simulink model "VehicleThermalSystemSizing"  (R2023b)
settings: Solver=daessc  StartTime=0  StopTime=600  FixedStep=0.2  MaxStep=1  RelTol=1e-3  AbsTol=1e-3
undefined symbols (not defined in the file): air_density, bulb, cabin_H, cabin_L, cabin_W, coolant_pipe_D, coolant_T_init, coolant_tank_volume, CoolingPower_kW, door_or_window_area, duct_W, evap_superheat_temp, inlet, pump_speed_max, refrigerant_massflowrate, RPM_Compressor_nominal, RPM_CondFan, RPM_EvapFan, T_cabin_init, T_set, tube_D, VolFlowrate_CondenserFan, VolFlowRate_CoolantRadiatorFan, VolFlowRate_EvapFan
libraries: fl_lib x128, nesl_utility x45, SimscapeFluids_lib x16, simulink_extras x9
(part 1 of 4)
Description:
  | Refrigeration Cycle (Air Conditioning)
settings Model: Creator=The MathWorks, Inc.  LastModifiedBy=fnae
settings SolverCC: AutoScaleAbsTol=off  AlgebraicLoopSolver=TrustRegion  MaxZcPerStep=1
settings DataIOCC: SaveFormat=StructureWithTime  ReturnWorkspaceOutputs=off
settings OptimizationCC: BlockReduction=off  BufferReuse=off  ReuseModelBlockBuffer=off
settings DebuggingCC: AlgebraicLoopMsg=none  SymbolicDimsDataTypeCodeGenerationDiagnostic=none
settings ModelReferenceCC: EnableRefExpFcnMdlSchedulingChecks=on
settings SFSimCC: CustomCodeUndefinedFunction=UseInterfaceOnly
settings RTWCC: DLArmComputeVersion=19.05
settings SimscapeCC: SimscapeLogType=all  SimscapeLogSimulationStatistics=on  SimscapeLogName=simlog_refrigeration  SimscapeLogLimitData=off  SimscapeLogDataHistory=10000  SimscapeOperatingPoint=operPoint
settings ExplorerConfigSet: SimMechanicsOpenEditorOnUpdate=off

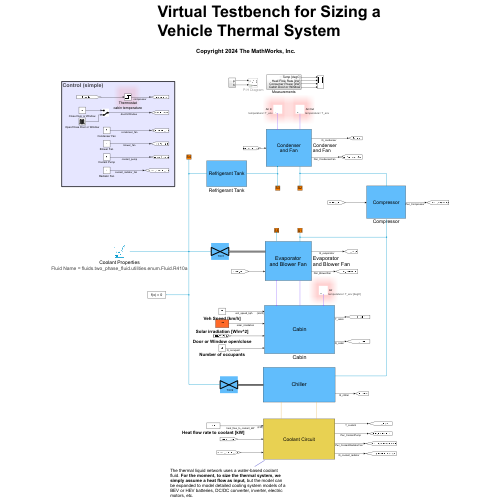
[thumbnail: Simulink's stored preview of the top-level diagram]
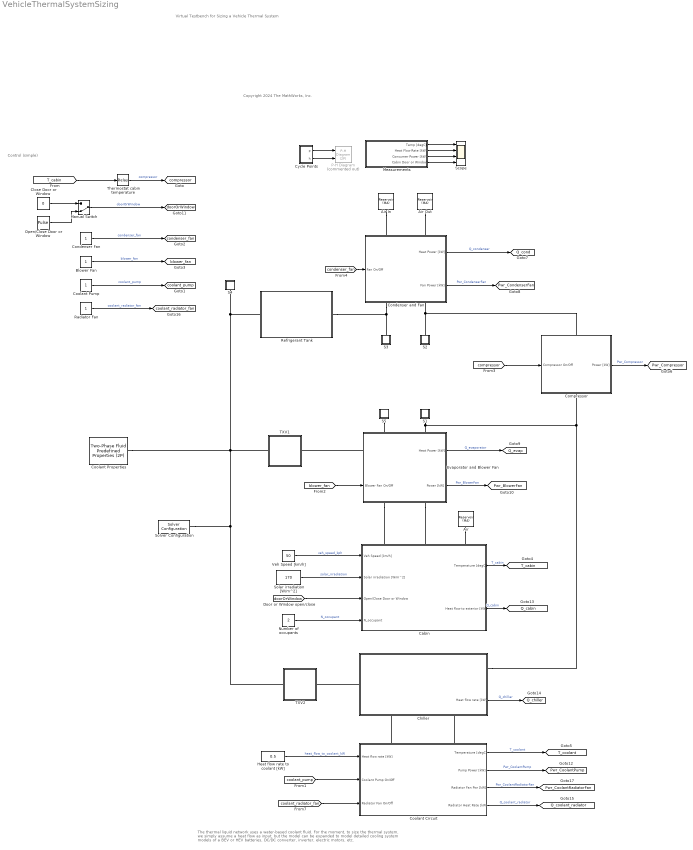
== system VehicleThermalSystemSizing ==
  note: The thermal liquid network uses a water-based coolant fluid. For the moment, to size the thermal system, we simply assume a heat flow as input, but the model can be expanded to model detailed cooling system models of a BEV or HEV batteries, DC/DC converter, inverter, electric motors, etc.
  note: Control (simple)
  note: Virtual Testbench for Sizing a Vehicle Thermal System
  note: Copyright 2024 The MathWorks, Inc.
  Air : fl_lib/Moist Air/Elements/Reservoir (MA)  pressure_spec=foundation.enum.pressure_spec.specified  reservoir_pressure=0.101325 MPa  temperature_spec=foundation.enum.temperature_spec.specified  reservoir_temperature=T_env degC  moisture_spec=foundation.enum.moisture_spec.relative_humidity  reservoir_RH=0.5  reservoir_x_w=0.01  reservoir_y_w=0.01  reservoir_HR=0.01  reservoir_Tw=287 K  trace_gas_spec=foundation.enum.trace_gas_spec.mole_fraction  reservoir_x_g=0.001  reservoir_y_g=0  RH_ws=1  area_A=duct_W^2 m^2
      settings: AttributesFormatString=temperature= %<reservoir_temperature> [%<reservoir_temperature_unit>]
  Air In : fl_lib/Moist Air/Elements/Reservoir (MA)  pressure_spec=foundation.enum.pressure_spec.specified  reservoir_pressure=0.101325 MPa  temperature_spec=foundation.enum.temperature_spec.specified  reservoir_temperature=T_env degC  moisture_spec=foundation.enum.moisture_spec.relative_humidity  reservoir_RH=0.5  reservoir_x_w=0.01  reservoir_y_w=0.01  reservoir_HR=0.01  reservoir_Tw=287 K  trace_gas_spec=foundation.enum.trace_gas_spec.mole_fraction  reservoir_x_g=0.001  reservoir_y_g=0  RH_ws=1  area_A=duct_W^2 m^2
      settings: AttributesFormatString=temperature= %<reservoir_temperature>
  Air Out : fl_lib/Moist Air/Elements/Reservoir (MA)  pressure_spec=foundation.enum.pressure_spec.specified  reservoir_pressure=0.101325 MPa  temperature_spec=foundation.enum.temperature_spec.specified  reservoir_temperature=T_env degC  moisture_spec=foundation.enum.moisture_spec.relative_humidity  reservoir_RH=0.5  reservoir_x_w=0.01  reservoir_y_w=0.01  reservoir_HR=0.01  reservoir_Tw=287 K  trace_gas_spec=foundation.enum.trace_gas_spec.mole_fraction  reservoir_x_g=0.001  reservoir_y_g=0  RH_ws=1  area_A=duct_W^2 m^2
      settings: AttributesFormatString=temperature= %<reservoir_temperature>
  Blower Fan : Constant  SampleTime=1
  Cabin : Subsystem
      settings: PortSchema="{\"entries\":[{\"content\":{\"sides\":[{\"content\":{\"connectorIds\":[\"In1\",\"In2\",\"In3\",\"In4\"]},\"type\":\"ConnectorPlacement.EquallySpacedRectSide\",\"uuid\":\"5cf57e4f-975f-4b0b-a8e8-bf86758a11fa\"},{\"content\":{\"connectorIds\":[\"Out1\",\"Out2\"],\"side\":\"RIGHT\"},\"type\":\"ConnectorPlacement.EquallySpacedRectSide\",\"uuid\":\"7f477a27-3a34-4ed6-85c3-331630c97133\"},{\"content\":{\"connectorIds\":[\"LConn1\",\"LConn2\",\"LConn3\"],\"side\":\"TOP\"},\"type\":\"ConnectorPlacement.EquallySpacedRectSide\",\"uuid\":\"743b5c17-84cf-4a2e-818e-c1a69eb195e5\"}]},\"type\":\"ConnectorPlacement.EquallySpacedConnector\",\"uuid\":\"4a6d6dd0-79df-4460-8879-70a258476fa5\"}],\"packageUris\":[\"http://schema.mathworks.com/mf0/Connector/R2020b\"],\"version\":\"1.0\"}"
      mask Display: disp(get_param(gcb, 'Name'));
  Chiller : Subsystem  Tag=PublishSubsystem
      settings: PortSchema="{\"entries\":[{\"content\":{\"sides\":[{\"content\":{\"connectorIds\":[\"Out1\",\"LConn1\"]},\"type\":\"ConnectorPlacement.EquallySpacedRectSide\",\"uuid\":\"684495fe-43ac-42d2-91f9-c1083f68d635\"},{\"content\":{\"connectorIds\":[\"RConn1\"],\"side\":\"RIGHT\"},\"type\":\"ConnectorPlacement.EquallySpacedRectSide\",\"uuid\":\"acb3d27a-41e1-4bfe-a4d6-36d5666e4ba3\"},{\"content\":{\"connectorIds\":[\"LConn2\",\"LConn3\"],\"side\":\"TOP\"},\"type\":\"ConnectorPlacement.EquallySpacedRectSide\",\"uuid\":\"cdadeb40-472c-4edb-91b8-a2216ea85c99\"},{\"content\":{\"side\":\"BOTTOM\"},\"type\":\"ConnectorPlacement.EquallySpacedRectSide\",\"uuid\":\"46a4312c-e637-44ea-bfb3-e887da9d9904\"}]},\"type\":\"ConnectorPlacement.EquallySpacedConnector\",\"uuid\":\"20e25167-e167-414a-8c66-12b35ae5ef5e\"}],\"packageUris\":[\"http://schema.mathworks.com/mf0/Connector/R2020b\"],\"version\":\"1.0\"}"
      mask Display: disp(get_param(gcb, 'Name'));
  Close Door or Window : Constant  Value=0  SampleTime=1
  Compressor : Subsystem
      settings: PortSchema="{\"entries\":[{\"content\":{\"sides\":[{\"content\":{\"connectorIds\":[\"LConn1\"]},\"type\":\"ConnectorPlacement.EquallySpacedRectSide\",\"uuid\":\"87497da4-7fcd-4c39-9d14-dd80365934db\"},{\"content\":{\"connectorIds\":[\"RConn1\"],\"side\":\"RIGHT\"},\"type\":\"ConnectorPlacement.EquallySpacedRectSide\",\"uuid\":\"c29b3d2b-7130-4a2f-8dcb-58b301edb84d\"},{\"content\":{\"connectorIds\":[\"In1\"],\"side\":\"TOP\"},\"type\":\"ConnectorPlacement.EquallySpacedRectSide\",\"uuid\":\"6b0e1579-3829-4056-a1f0-26424a36bca1\"},{\"content\":{\"connectorIds\":[\"Out1\"],\"side\":\"BOTTOM\"},\"type\":\"ConnectorPlacement.EquallySpacedRectSide\",\"uuid\":\"6b49380d-e724-4e3a-86e0-6bc21724e354\"}]},\"type\":\"ConnectorPlacement.EquallySpacedConnector\",\"uuid\":\"16d6c8a7-8265-44ec-91d1-631bbb83e0af\"}],\"packageUris\":[\"http://schema.mathworks.com/mf0/Connector/R2020b\"],\"version\":\"1.0\"}"
      mask Display: disp(get_param(gcb, 'Name'));
  Condenser and Fan : Subsystem
      settings: PortSchema="{\"entries\":[{\"content\":{\"sides\":[{\"content\":{\"connectorIds\":[\"LConn1\",\"LConn2\"]},\"type\":\"ConnectorPlacement.EquallySpacedRectSide\",\"uuid\":\"94f743b0-016e-4f6c-ba37-cd5c9e5decb1\"},{\"content\":{\"connectorIds\":[\"RConn1\",\"RConn2\"],\"side\":\"RIGHT\"},\"type\":\"ConnectorPlacement.EquallySpacedRectSide\",\"uuid\":\"4e78d493-e8a5-489f-9c9b-6c9134237572\"},{\"content\":{\"connectorIds\":[\"In1\"],\"side\":\"TOP\"},\"type\":\"ConnectorPlacement.EquallySpacedRectSide\",\"uuid\":\"0b95dc75-9fe3-4b9e-8dc0-c99924a5b683\"},{\"content\":{\"connectorIds\":[\"Out1\",\"Out2\"],\"side\":\"BOTTOM\"},\"type\":\"ConnectorPlacement.EquallySpacedRectSide\",\"uuid\":\"eea3e702-1cf4-4504-9501-89c4531d7134\"}]},\"type\":\"ConnectorPlacement.EquallySpacedConnector\",\"uuid\":\"0b0f7158-6d74-402a-9204-25c9a3fd4099\"}],\"packageUris\":[\"http://schema.mathworks.com/mf0/Connector/R2020b\"],\"version\":\"1.0\"}"
      mask Display: disp(get_param(gcb, 'Name'));
  Condenser Fan : Constant  SampleTime=1
  Coolant Circuit : Subsystem
      settings: PortSchema="{\"entries\":[{\"content\":{\"sides\":[{\"content\":{\"connectorIds\":[\"In1\",\"In2\",\"In3\"]},\"type\":\"ConnectorPlacement.EquallySpacedRectSide\",\"uuid\":\"61b3bd2b-efba-48b8-bc1e-7d5fd1f93ea8\"},{\"content\":{\"connectorIds\":[\"Out1\",\"Out2\",\"Out3\",\"Out4\"],\"side\":\"RIGHT\"},\"type\":\"ConnectorPlacement.EquallySpacedRectSide\",\"uuid\":\"116770ca-4665-4fbe-8ef7-14ad65bf6363\"},{\"content\":{\"connectorIds\":[\"LConn1\",\"LConn2\"],\"side\":\"TOP\"},\"type\":\"ConnectorPlacement.EquallySpacedRectSide\",\"uuid\":\"8588f2a2-4124-40f5-9c68-b1b3344e047c\"}]},\"type\":\"ConnectorPlacement.EquallySpacedConnector\",\"uuid\":\"af351b75-e118-4ad1-8604-555a25a7fec0\"}],\"packageUris\":[\"http://schema.mathworks.com/mf0/Connector/R2020b\"],\"version\":\"1.0\"}"
      mask Display: disp(get_param(gcb, 'Name'));
  Coolant Properties : SimscapeFluids_lib/Two-Phase Fluid/Utilities/Two-Phase Fluid Predefined Properties (2P)  fluid=fluids.two_phase_fluid.utilities.enum.Fluid.R410a  p_atm=0.101325 MPa  properties_range_check=simscape.enum.assert.action.error  q_rev=0.01 Pa
      settings: AttributesFormatString=Fluid Name = %<fluid>
  Coolant Pump : Constant  SampleTime=1
  Cycle Points : Subsystem
  Evaporator and Blower Fan : Subsystem
      settings: PortSchema="{\"entries\":[{\"content\":{\"sides\":[{\"content\":{\"connectorIds\":[\"LConn1\",\"LConn2\"]},\"type\":\"ConnectorPlacement.EquallySpacedRectSide\",\"uuid\":\"94f743b0-016e-4f6c-ba37-cd5c9e5decb1\"},{\"content\":{\"connectorIds\":[\"RConn1\",\"RConn2\"],\"side\":\"RIGHT\"},\"type\":\"ConnectorPlacement.EquallySpacedRectSide\",\"uuid\":\"4e78d493-e8a5-489f-9c9b-6c9134237572\"},{\"content\":{\"connectorIds\":[\"LConn3\",\"In1\"],\"side\":\"TOP\"},\"type\":\"ConnectorPlacement.EquallySpacedRectSide\",\"uuid\":\"0b95dc75-9fe3-4b9e-8dc0-c99924a5b683\"},{\"content\":{\"connectorIds\":[\"Out1\",\"Out2\"],\"side\":\"BOTTOM\"},\"type\":\"ConnectorPlacement.EquallySpacedRectSide\",\"uuid\":\"3125a7ac-4364-4843-9f9a-28cc842c280f\"}]},\"type\":\"ConnectorPlacement.EquallySpacedConnector\",\"uuid\":\"0b0f7158-6d74-402a-9204-25c9a3fd4099\"}],\"packageUris\":[\"http://schema.mathworks.com/mf0/Connector/R2020b\"],\"version\":\"1.0\"}"
      mask Display: disp(get_param(gcb, 'Name'));
  Heat flow rate to coolant [kW] : Constant  Value=0.5  SampleTime=1
  Manual Switch : ManualSwitch  CurrentSetting=0
  Measurements : Subsystem
  Number of occupants : Constant  Value=2  SampleTime=1
  Open/Close Door or Window : DiscretePulseGenerator  PulseType=Time based  Period=300  PulseWidth=5
  P-H Diagram : SimscapeFluids_lib/Two-Phase Fluid/Utilities/P-H Diagram (2P)  Commented=on
  Radiator Fan : Constant  SampleTime=1
  Refrigerant Tank : Subsystem
      mask Display: disp(get_param(gcb, 'Name'));
  S1 : Subsystem
      mask Display: disp(get_param(gcb, 'Name'))
  S2 : Subsystem
      mask Display: disp(get_param(gcb, 'Name'))
  S3 : Subsystem
      settings: PortSchema="{\"entries\":[{\"content\":{\"sides\":[{\"content\":{\"connectorIds\":[]},\"type\":\"ConnectorPlacement.EquallySpacedRectSide\",\"uuid\":\"16f002de-4636-401c-8be6-20698decbc91\"},{\"content\":{\"connectorIds\":[],\"side\":\"RIGHT\"},\"type\":\"ConnectorPlacement.EquallySpacedRectSide\",\"uuid\":\"76477188-11a3-4efa-a92e-0d269d480ac3\"},{\"content\":{\"connectorIds\":[],\"side\":\"TOP\"},\"type\":\"ConnectorPlacement.EquallySpacedRectSide\",\"uuid\":\"05fe64e4-9858-4712-a671-6ec27cab8615\"},{\"content\":{\"connectorIds\":[\"RConn1\"],\"side\":\"BOTTOM\"},\"type\":\"ConnectorPlacement.EquallySpacedRectSide\",\"uuid\":\"ddad7bbe-c900-450c-9863-e8fdc2274286\"}]},\"type\":\"ConnectorPlacement.EquallySpacedConnector\",\"uuid\":\"12bdef6d-66b8-4c10-9167-065994fcb3b8\"}],\"packageUris\":[\"http://schema.mathworks.com/mf0/Connector/R2020b\"],\"version\":\"1.0\"}"
      mask Display: disp(get_param(gcb, 'Name'))
  S4 : Subsystem
      mask Display: disp(get_param(gcb, 'Name'))
  S5 : Subsystem
      mask Display: disp(get_param(gcb, 'Name'))
  Scope : Scope  NumInputPorts=4
  Solar irradiation [W/m^2] : Constant  Value=170
  Solver Configuration : nesl_utility/Solver Configuration  PhysicalDomain=network_engine_domain  SubClassName=solver  LeftPortType=input  RightPortType=generic  Tones=[]  Harmonics=[]  SimulateNoise=off  Profile=off  UseLocalSampling=off  EnableSwitchedLinearOptims=on  FrequencyDomain=off  UseCCode=off  RelTol=0.001  AbsTol=0.001  MinStep=1e-09  ToWorkspace=off  RevertToSquareIcSolve=off  NumHomotopyIterations=100  PhasorMode=off  PhasorModeNumHarmonics=1  ConsistencySolver=NEWTON_XTOL_AFTER_FTOL  IndexReductionMethod=DerivativeReplacement  DoDC=off  ResidualTolerance=1e-6  ConsistencyTolSource=GLOBAL  ConsistencyAbsTol=0.001  ConsistencyRelTol=0.001  ConsistencyTolFactor=0.001  UseLocalSolver=off  LocalSolverChoice=NE_BACKWARD_EULER_ADVANCER  ResolveIndetEquations=on  FunctionEvalNumThread=1  LocalSolverSampleTime=0.01  DoFixedCost=off  MaxNonlinIter=100  MaxModeIter=10  ComputeImpulses=off  ImpulseIterations=2  LinearAlgebra=auto  LinearAlgebraNumThread=0  EquationFormulation=NE_TIME_EF  DelaysMemoryBudget=1024  AutomaticFiltering=on  FilteringTimeConstant=0.001  PartitionStorageMethod=AS_NEEDED  PartitionMemoryBudget=1024  PartitionMethod=ROBUST  MultibodyUseLocalSolver=off  MultibodyLocalSolverChoice=ODE1  MultibodyLocalSolverSampleTime=0.001
  TXV1 : Subsystem  Tag=PublishSubsystem
      mask Display:
      | color('white')
      | plot(100, 100)
      | plot(-100, -100)
      | color('black')
      | 
      | plot([0 -100 -100 0], [0 50 -50 0])
      | plot([0 100 100 0], [0 50 -50 0])
      | 
      | text(-50,60,get_param(gcb, 'Name'))
  TXV2 : Subsystem  Tag=PublishSubsystem
      mask Display:
      | color('white')
      | plot(100, 100)
      | plot(-100, -100)
      | color('black')
      | 
      | plot([0 -100 -100 0], [0 50 -50 0])
      | plot([0 100 100 0], [0 50 -50 0])
      | 
      | text(-50,60,get_param(gcb, 'Name'))
  Thermostat cabin temperature : Relay  OnSwitchValue=T_set + 1  OffSwitchValue=T_set  ZeroCross=off
  Veh Speed [km/h] : Constant  Value=50  SampleTime=1
  tag scope: Pwr_BlowerFan=global, Pwr_Compressor=global, Pwr_CondenserFan=global, Pwr_CoolantPump=global, Pwr_CoolantRadiatorFan=global, Q_cabin=global, Q_chiller=global, Q_cond=global, Q_coolant_radiator=global, Q_evap=global, T_cabin=global, T_coolant=global, blower_fan=global, compressor=global, condenser_fan=global, coolant_pump=global, coolant_radiator_fan=global, doorOrWindow=global
  wires:
  Cycle Points/1(p) -> P-H Diagram/1
  Cycle Points/2(h) -> P-H Diagram/2
  Measurements/1(Temp [degC]) -> Scope/1
  Measurements/2(Heat Flow Rate [kW]) -> Scope/2
  Measurements/3(Consumer Power [kW]) -> Scope/3
  Measurements/4(Cabin Door or Window) -> Scope/4
  [T_cabin] -> Thermostat cabin temperature/1
  [condenser_fan] -> Condenser and Fan/1(Fan On/Off)
  Condenser Fan/1 -> [condenser_fan]  "condenser_fan"
  [compressor] -> Compressor/1(Compressor On/Off)
  Blower Fan/1 -> [blower_fan]  "blower_fan"
  [blower_fan] -> Evaporator and Blower Fan/1(Blower Fan On/Off)
  Veh Speed [km/h]/1 -> Cabin/1(Veh Speed [km/h])  "veh_speed_kph"
  Solar irradiation [W/m^2]/1 -> Cabin/2(Solar irradiation [W/m^2])  "solar_irradiation"
  Coolant Pump/1 -> [coolant_pump]  "coolant_pump"
  Cabin/1(Temperature [degC]) -> [T_cabin]  "T_cabin"
  Compressor/1(Power [kW]) -> [Pwr_Compressor]  "Pwr_Compressor"
  Evaporator and Blower Fan/1(Heat Power [kW]) -> [Q_evap]  "Q_evaporator"
  Evaporator and Blower Fan/2(Power [kW]) -> [Pwr_BlowerFan]  "Pwr_BlowerFan"
  Manual Switch/1 -> [doorOrWindow]  "doorOrWindow"
  [doorOrWindow] -> Cabin/3(Open/Close Door or Window)
  Cabin/2(Heat flow to exterior [kW]) -> [Q_cabin]  "Q_cabin"
  Condenser and Fan/2(Fan Power [kW]) -> [Pwr_CondenserFan]  "Pwr_CondenserFan"
  Condenser and Fan/1(Heat Power [kW]) -> [Q_cond]  "Q_condenser"
  Radiator Fan/1 -> [coolant_radiator_fan]  "coolant_radiator_fan"
  Thermostat cabin temperature/1 -> [compressor]  "compressor"
  Chiller/1(Heat flow rate [kW]) -> [Q_chiller]  "Q_chiller"
  Heat flow rate to coolant [kW]/1 -> Coolant Circuit/1(Heat flow rate [kW])  "heat_flow_to_coolant_kW"
  Coolant Circuit/4(Radiator Heat Rate [kW]) -> [Q_coolant_radiator]  "Q_coolant_radiator"
  Coolant Circuit/2(Pump Power [kW]) -> [Pwr_CoolantPump]  "Pwr_CoolantPump"
  [coolant_pump] -> Coolant Circuit/2(Coolant Pump On/Off)
  Coolant Circuit/1(Temperature [degC]) -> [T_coolant]  "T_coolant"
  [coolant_radiator_fan] -> Coolant Circuit/3(Radiator Fan On/Off)
  Coolant Circuit/3(Radiator Fan Pwr [kW]) -> [Pwr_CoolantRadiatorFan]  "Pwr_CoolantRadiatorFan"
  Close Door or Window/1 -> Manual Switch/1
  Open/Close Door or Window/1 -> Manual Switch/2
  Number of occupants/1 -> Cabin/4(N_occupant)  "N_occupant"
  connections:
  Condenser and Fan/RConn1 -- Refrigerant Tank/RConn1 -- S3/RConn1
  S5/LConn1 -- Evaporator and Blower Fan/LConn1
  Condenser and Fan/RConn2 -- Compressor/RConn1 -- S2/LConn1
  Air In/LConn1 -- Condenser and Fan/LConn1
  Air Out/LConn1 -- Condenser and Fan/LConn2
  Evaporator and Blower Fan/LConn3 -- TXV1/LConn1
  TXV1/RConn1 -- TXV2/RConn1 -- Solver Configuration/RConn1 -- S4/LConn1 -- Refrigerant Tank/LConn1 -- Coolant Properties/RConn1
  Evaporator and Blower Fan/RConn2 -- Cabin/LConn2
  Evaporator and Blower Fan/RConn1 -- Cabin/LConn1
  Air/LConn1 -- Cabin/LConn3
  S1/LConn1 -- Chiller/LConn1 -- Compressor/LConn1 -- Evaporator and Blower Fan/LConn2
  Chiller/RConn1 -- TXV2/LConn1
  Coolant Circuit/LConn1 -- Chiller/LConn3
  Coolant Circuit/LConn2 -- Chiller/LConn2

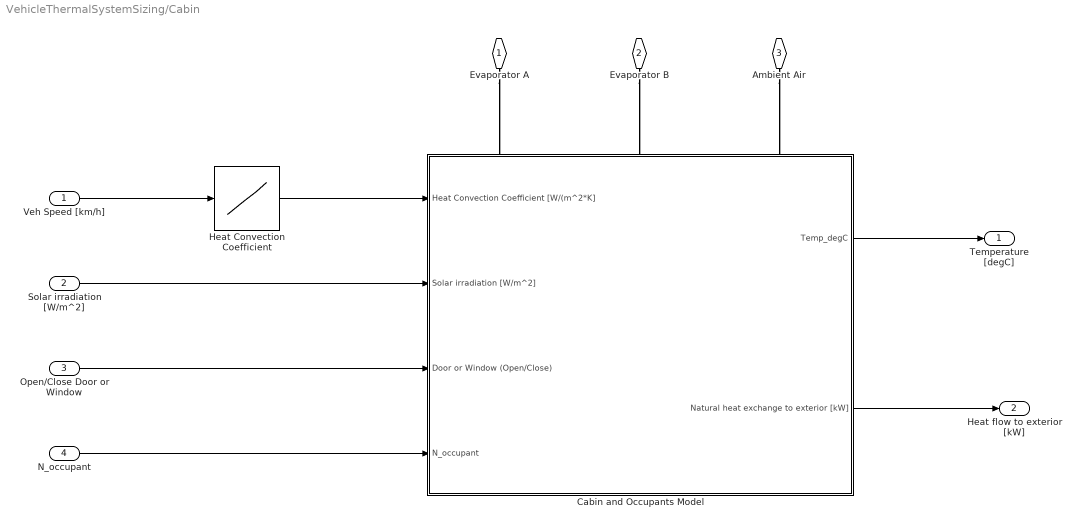
== system VehicleThermalSystemSizing/Cabin ==
  Veh Speed [km/h] : Inport  Unit=km/hour
  Solar irradiation [W/m^2] : Inport  Port=2
  Open/Close Door or Window : Inport  Port=3
  N_occupant : Inport  Port=4
  Cabin and Occupants Model : Subsystem  Tag=PublishSubsystem  mask(Cooling Volume){coolingBox_L=cabin_L, coolingBox_W=cabin_W, coolingBox_H=cabin_H, T_cabin_init_degC=T_cabin_init, door_or_window_area=door_or_window_area}
      mask prompts: coolingBox_L "Length (m)"; coolingBox_W "Width (m)"; coolingBox_H "Height (m)"; T_cabin_init_degC "Initial inside temperature (degC)"; door_or_window_area "Door area (m^2)"
      settings: PortSchema="{\"entries\":[{\"content\":{\"sides\":[{\"content\":{\"connectorIds\":[\"In1\",\"In2\",\"In3\",\"In4\"]},\"type\":\"ConnectorPlacement.EquallySpacedRectSide\",\"uuid\":\"e1f7673a-ae09-4e38-a748-d03f3a89f634\"},{\"content\":{\"connectorIds\":[\"Out1\",\"Out2\"],\"side\":\"RIGHT\"},\"type\":\"ConnectorPlacement.EquallySpacedRectSide\",\"uuid\":\"e2c59df4-5a81-4f6b-ab06-631ef800c0b1\"},{\"content\":{\"connectorIds\":[\"LConn1\",\"LConn2\",\"LConn3\"],\"side\":\"TOP\"},\"type\":\"ConnectorPlacement.EquallySpacedRectSide\",\"uuid\":\"19dd88a8-04e0-4296-a227-9de66059cdf8\"}]},\"type\":\"ConnectorPlacement.EquallySpacedConnector\",\"uuid\":\"cfca4f7e-9c0e-462b-910e-b09b0fceba6e\"}],\"packageUris\":[\"http://schema.mathworks.com/mf0/Connector/R2020b\"],\"version\":\"1.0\"}"
      settings: AttributesFormatString=|
      | Length= %<coolingBox_L>
      | Width= %<coolingBox_W>
      | Height= %<coolingBox_H>
      | Initial Temp= %<T_cabin_init_degC>
  Heat Convection Coefficient : Lookup_n-D  NumberOfTableDimensions=1  BreakpointsForDimension1=[0 5 10]  Table=[1 50 100]  InternalRulePriority=Speed  RndMeth=Simplest
  Evaporator A : PMIOPort  Side=Left
  Evaporator B : PMIOPort  Port=2  Side=Left
  Ambient Air : PMIOPort  Port=3  Side=Left
  Temperature [degC] : Outport
  Heat flow to exterior [kW] : Outport  Port=2
  wires:
  Veh Speed [km/h]/1 -> Heat Convection Coefficient/1
  Heat Convection Coefficient/1 -> Cabin and Occupants Model/1(Heat Convection Coefficient [W/(m^2*K])
  Solar irradiation [W/m^2]/1 -> Cabin and Occupants Model/2(Solar irradiation [W/m^2])
  Cabin and Occupants Model/1(Temp_degC) -> Temperature [degC]/1
  Open/Close Door or Window/1 -> Cabin and Occupants Model/3(Door or Window (Open/Close))
  Cabin and Occupants Model/2(Natural heat exchange to exterior [kW]) -> Heat flow to exterior [kW]/1
  N_occupant/1 -> Cabin and Occupants Model/4(N_occupant)
  connections:
  Evaporator B/RConn1 -- Cabin and Occupants Model/LConn2
  Evaporator A/RConn1 -- Cabin and Occupants Model/LConn1
  Ambient Air/RConn1 -- Cabin and Occupants Model/LConn3

== system VehicleThermalSystemSizing/Chiller ==
  note: Heat exchanger (system-level model) that lets the refrigerant absorb heat from the coolant.This way the coolant (water glycol) from the battery is cooled and heats the refrigerant (R410a)
  note: This is a model of a chiller that uses two-phase refrigeration circuit to cool a thermal liquid network. The thermal liquid network uses a water-based coolant fluid and the model can be expanded to model cooling of a BEV or HEV battery, DC/DC converter, inverter, electric motors, etc.
  Chiller (System-Level) : SimscapeFluids_lib/Fluid Network Interfaces/Heat Exchangers/System-Level Condenser Evaporator (2P-TL)  flow_arrangement=fluids.interfaces.heat_exchangers.enum.SystemLevelFlowArrangement2PTL.Cross  wall_thermal_mass=false  mass_wall=1 kg  cp_wall=490 J/(K*kg)  nominal_init_wall=true  T_wall_init=293.15 K  area_A1=pi*tube_D^2/4 m^2  area_B1=pi*tube_D^2/4 m^2  area_A2=pi*tube_D^2/4 m^2  area_B2=pi*tube_D^2/4 m^2  operating_condition_2P=fluids.interfaces.heat_exchangers.enum.SystemLevelOperatingCondition2PTL.Evaporator  mdot_nominal_2P=0.5*refrigerant_massflowrate kg/s  delta_p_nominal_2P=0.01 MPa  pressure_spec_cond_2P=fluids.interfaces.heat_exchangers.enum.SystemLevelPressureSpecCondenser2P.InletPressure  pressure_spec_evap_2P=fluids.interfaces.heat_exchangers.enum.SystemLevelPressureSpecEvaporator2P.EvaporatingTemperature  p_in_nominal_2P=1 MPa  T_cond_nominal_2P=313.15 K  T_evap_nominal_2P=nominal_evap_temp degC  inlet_spec_2P=fluids.interfaces.heat_exchangers.enum.SystemLevelInletSpec2P.Enthalpy  T_in_nominal_2P=333.15 K  h_in_nominal_2P=evap_inlet_enthalpy kJ/kg  x_in_nominal_2P=1  capacity_spec_2P=fluids.interfaces.heat_exchangers.enum.SystemLevelCapacitySpec.OutletCondition  Q_nominal=0.1 kW  outlet_spec_cond_2P=fluids.interfaces.heat_exchangers.enum.SystemLevelOutletSpecCondenser2P.Enthalpy  outlet_spec_evap_2P=fluids.interfaces.heat_exchangers.enum.SystemLevelOutletSpecEvaporator2P.Superheating  delta_T_sub_nominal_2P=5 deltaK  delta_T_sup_nominal_2P=evap_superheat_temp deltaK  h_out_nominal_2P=250 kJ/kg  x_out_nominal_2P=0  volume_2P=0.001 m^3  nominal_init_2P=false  energy_spec_2P=foundation.enum.energy_spec.enthalpy  p_init_2P=evap_inlet_p MPa  T_init_2P=293.15 K  x_init_2P=0.5  alpha_init_2P=0.5  h_init_2P=evap_inlet_enthalpy kJ/kg  u_init_2P=1500 kJ/kg  mdot_nominal_TL=pump_nominal_massflowrate kg/s  delta_p_nominal_TL=0.01 MPa  p_in_nominal_TL=coolant_p_init MPa  T_in_nominal_TL=coolant_T_init degC  volume_TL=0.001 m^3  nominal_init_TL=true  p_init_TL=0.101325 MPa  T_init_TL=293.15 K  a_liq_2P=0.023  a_mix_2P=0.005  a_vap_2P=0.023  b_2P=0.8  c_2P=0.33  a_TL=0.023  b_TL=0.8  c_TL=0.33
      settings: InternalSimscapePortConfiguration="{\"Bottom\":[],\"Left\":[{\"id\":\"A1\",\"label\":\"A1\",\"type\":\"foundation.two_phase_fluid.two_phase_fluid\"},{\"id\":\"B1\",\"label\":\"B1\",\"type\":\"foundation.two_phase_fluid.two_phase_fluid\"}],\"Right\":[{\"id\":\"A2\",\"label\":\"A2\",\"type\":\"foundation.thermal_liquid.thermal_liquid\"},{\"id\":\"B2\",\"label\":\"B2\",\"type\":\"foundation.thermal_liquid.thermal_liquid\"}],\"Top\":[{\"id\":\"Q1\",\"label\":\"Q1\",\"type\":\"output\"},{\"id\":\"Q2\",\"label\":\"Q2\",\"type\":\"output\"}]}"
  PS-Simulink Converter1 : nesl_utility/PS-Simulink Converter  PhysicalDomain=network_engine_domain  SubClassName=ps_output  LeftPortType=input  RightPortType=output  PseudoPeriodic=off  Frequencies=[]  VectorFormat=inherit  Unit=kW  AffineConversion=off
  Simscape Bus : SimscapeBus  HierarchyStrings=bulb;inlet
  To Compressor : PMIOPort  Side=Left
  C : PMIOPort  Port=2  Side=Left
  D : PMIOPort  Port=3  Side=Left
  To TXV : PMIOPort  Port=4  Side=Right
  Heat flow rate [kW] : Outport
  wires:
  PS-Simulink Converter1/1 -> Heat flow rate [kW]/1
  connections:
  To TXV/RConn1 -- Simscape Bus/RConn1
  Simscape Bus/LConn1 -- Chiller (System-Level)/LConn2 -- To Compressor/RConn1
  Simscape Bus/LConn2 -- Chiller (System-Level)/LConn1
  Chiller (System-Level)/RConn1 -- C/RConn1
  Chiller (System-Level)/RConn2 -- D/RConn1
  PS-Simulink Converter1/LConn1 -- Chiller (System-Level)/LConn3

== system VehicleThermalSystemSizing/Compressor ==
  Compressor On/Off : Inport
  Compressor : Subsystem  Variant=on  VariantControlMode=label  LabelModeActiveChoice=Compressor_detailed
  Evap Outlet : PMIOPort  Side=Left
  Condenser Inlet : PMIOPort  Port=2  Side=Right
  Power [kW] : Outport
  wires:
  Compressor On/Off/1 -> Compressor/1(Compressor On/Off)
  Compressor/1(Power [kW]) -> Power [kW]/1
  connections:
  Evap Outlet/RConn1 -- Compressor/LConn1
  Condenser Inlet/RConn1 -- Compressor/RConn1

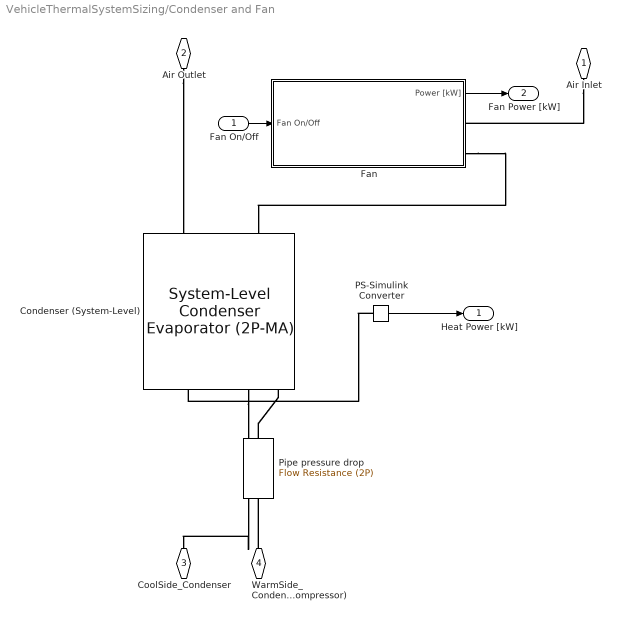
== system VehicleThermalSystemSizing/Condenser and Fan ==
  Fan On/Off : Inport
  Condenser (System-Level) : SimscapeFluids_lib/Fluid Network Interfaces/Heat Exchangers/System-Level Condenser Evaporator (2P-MA)  flow_arrangement=fluids.interfaces.heat_exchangers.enum.SystemLevelFlowArrangement2PMA.Cross  wall_thermal_mass=simscape.enum.onoff.off  mass_wall=1 kg  cp_wall=490 J/(K*kg)  nominal_init_wall=true  T_wall_init=293.15 K  area_A1=pi*tube_D^2/4 m^2  area_B1=pi*tube_D^2/4 m^2  area_A2=duct_W^2 m^2  area_B2=duct_W^2 m^2  operating_condition_2P=fluids.interfaces.heat_exchangers.enum.SystemLevelOperatingCondition2PMA.Condenser  mdot_nominal_2P=refrigerant_massflowrate kg/s  delta_p_nominal_2P=0.01 MPa  pressure_spec_cond_2P=fluids.interfaces.heat_exchangers.enum.SystemLevelPressureSpecCondenser2P.CondensingTemperature  pressure_spec_evap_2P=fluids.interfaces.heat_exchangers.enum.SystemLevelPressureSpecEvaporator2P.InletPressure  p_in_nominal_2P=1 MPa  T_cond_nominal_2P=nominal_condens_temp degC  T_evap_nominal_2P=243.15 K  inlet_spec_2P=fluids.interfaces.heat_exchangers.enum.SystemLevelInletSpec2P.Temperature  T_in_nominal_2P=condenser_inlet_temp degC  h_in_nominal_2P=440 kJ/kg  x_in_nominal_2P=1  capacity_spec_2P=fluids.interfaces.heat_exchangers.enum.SystemLevelCapacitySpec.OutletCondition  Q_nominal=0.1 kW  outlet_spec_cond_2P=fluids.interfaces.heat_exchangers.enum.SystemLevelOutletSpecCondenser2P.Subcooling  outlet_spec_evap_2P=fluids.interfaces.heat_exchangers.enum.SystemLevelOutletSpecEvaporator2P.Enthalpy  delta_T_sub_nominal_2P=condenser_subcooling_temp deltaK  delta_T_sup_nominal_2P=5 deltaK  h_out_nominal_2P=condenser_inlet_p kJ/kg  x_out_nominal_2P=0  volume_2P=0.001 m^3  nominal_init_2P=true  energy_spec_2P=foundation.enum.energy_spec.enthalpy  p_init_2P=condenser_inlet_p MPa  T_init_2P=refrig_T_init degC  x_init_2P=0.5  alpha_init_2P=0.5  h_init_2P=condenser_inlet_enthalpy kJ/kg  u_init_2P=1500 kJ/kg  mdot_nominal_MA=evap_air_massflowrate kg/s  delta_p_nominal_MA=200 Pa  p_in_nominal_MA=0.101325 MPa  T_in_nominal_MA=T_set degC  inlet_moisture_spec_MA=foundation.enum.moisture_spec.relative_humidity  RH_in_nominal_MA=0.5  x_w_in_nominal_MA=0.01  y_w_in_nominal_MA=0.01  HR_in_nominal_MA=0.01  inlet_trace_gas_spec_MA=foundation.enum.trace_gas_spec.mole_fraction  x_g_in_nominal_MA=0.001  y_g_in_nominal_MA=0  volume_MA=0.15 m^3  nominal_init_MA=true  p_init_MA=moist_air_p_init MPa  T_init_MA=moist_air_T_init degC  moisture_spec_MA=foundation.enum.moisture_spec.relative_humidity  RH_init_MA=moist_air_RH_init  x_w_init_MA=0.01  y_w_init_MA=0.01  HR_init_MA=0.01  trace_gas_spec_MA=foundation.enum.trace_gas_spec.mass_fraction  x_g_init_MA=0.001  y_g_init_MA=0.001  RH_ws_MA=1  a_liq_2P=0.023  a_mix_2P=0.005  a_vap_2P=0.023  b_2P=0.8  c_2P=0.33  a_MA=0.023  b_MA=0.8  c_MA=0.33
      settings: InternalSimscapePortConfiguration="{\"Bottom\":[],\"Left\":[{\"id\":\"A1\",\"label\":\"A1\",\"type\":\"foundation.two_phase_fluid.two_phase_fluid\"},{\"id\":\"B1\",\"label\":\"B1\",\"type\":\"foundation.two_phase_fluid.two_phase_fluid\"}],\"Right\":[{\"id\":\"A2\",\"label\":\"A2\",\"type\":\"foundation.moist_air.moist_air\"},{\"id\":\"B2\",\"label\":\"B2\",\"type\":\"foundation.moist_air.moist_air\"}],\"Top\":[{\"id\":\"Q1\",\"label\":\"Q1\",\"type\":\"output\"},{\"id\":\"Q2\",\"label\":\"Q2\",\"type\":\"output\"},{\"id\":\"W\",\"label\":\"W\",\"type\":\"output\"}]}"
  Fan : Subsystem  Variant=on  VariantControlMode=label  LabelModeActiveChoice=Fan_simple
  PS-Simulink Converter : nesl_utility/PS-Simulink Converter  PhysicalDomain=network_engine_domain  SubClassName=ps_output  LeftPortType=input  RightPortType=output  PseudoPeriodic=off  Frequencies=[]  VectorFormat=inherit  Unit=kW  AffineConversion=off
  Pipe pressure drop : fl_lib/Two-Phase Fluid/Elements/Flow Resistance (2P)  delta_p_nominal=100 Pa  mdot_nominal=refrigerant_massflowrate kg/s  v_nominal=0 m^3/kg  area=pi*tube_D^2/4 m^2  laminar_fraction=1e-3
      settings: InternalSimscapePortConfiguration="{\"Bottom\":[],\"Left\":[{\"id\":\"A\",\"label\":\"A\",\"type\":\"foundation.two_phase_fluid.two_phase_fluid\"}],\"Right\":[{\"id\":\"B\",\"label\":\"B\",\"type\":\"foundation.two_phase_fluid.two_phase_fluid\"}],\"Top\":[]}"
  Air Inlet : PMIOPort  Side=Left
  Air Outlet : PMIOPort  Port=2  Side=Left
  CoolSide_Condenser : PMIOPort  Port=3  Side=Right
  WarmSide_Condenser (from Compressor) : PMIOPort  Port=4  Side=Right
  Heat Power [kW] : Outport
  Fan Power [kW] : Outport  Port=2
  wires:
  Fan On/Off/1 -> Fan/1(Fan On/Off)
  Fan/1(Power [kW]) -> Fan Power [kW]/1
  PS-Simulink Converter/1 -> Heat Power [kW]/1
  connections:
  Air Outlet/RConn1 -- Condenser (System-Level)/RConn2
  PS-Simulink Converter/LConn1 -- Condenser (System-Level)/LConn4
  WarmSide_Condenser (from Compressor)/RConn1 -- Pipe pressure drop/LConn1
  Condenser (System-Level)/LConn2 -- CoolSide_Condenser/RConn1
  Air Inlet/RConn1 -- Fan/RConn1
  Fan/RConn2 -- Condenser (System-Level)/RConn1
  Pipe pressure drop/RConn1 -- Condenser (System-Level)/LConn1

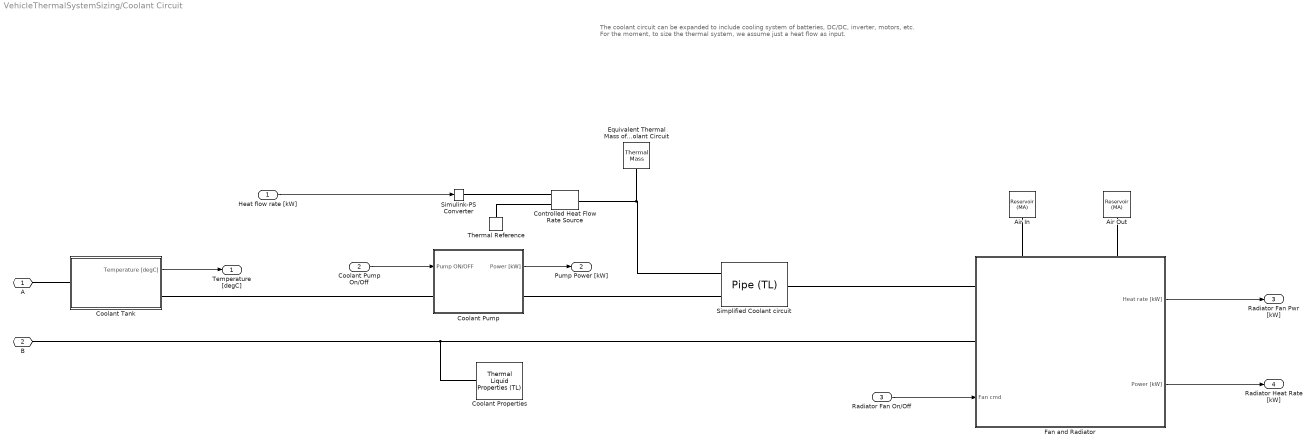
== system VehicleThermalSystemSizing/Coolant Circuit ==
  note: The coolant circuit can be expanded to include cooling system of batteries, DC/DC, inverter, motors, etc.
      | For the moment, to size the thermal system, we assume just a heat flow as input.
  Heat flow rate [kW] : Inport  Unit=kW
  Coolant Pump On/Off : Inport  Port=2
  Radiator Fan On/Off : Inport  Port=3
  Air In : fl_lib/Moist Air/Elements/Reservoir (MA)  pressure_spec=foundation.enum.pressure_spec.specified  reservoir_pressure=0.101325 MPa  temperature_spec=foundation.enum.temperature_spec.specified  reservoir_temperature=T_env degC  moisture_spec=foundation.enum.moisture_spec.relative_humidity  reservoir_RH=0.5  reservoir_x_w=0.01  reservoir_y_w=0.01  reservoir_HR=0.01  reservoir_Tw=287 K  trace_gas_spec=foundation.enum.trace_gas_spec.mole_fraction  reservoir_x_g=0.001  reservoir_y_g=0  RH_ws=1  area_A=duct_W^2 m^2
      settings: AttributesFormatString=temperature= %<reservoir_temperature>
  Air Out : fl_lib/Moist Air/Elements/Reservoir (MA)  pressure_spec=foundation.enum.pressure_spec.specified  reservoir_pressure=0.101325 MPa  temperature_spec=foundation.enum.temperature_spec.specified  reservoir_temperature=T_env degC  moisture_spec=foundation.enum.moisture_spec.relative_humidity  reservoir_RH=0.5  reservoir_x_w=0.01  reservoir_y_w=0.01  reservoir_HR=0.01  reservoir_Tw=287 K  trace_gas_spec=foundation.enum.trace_gas_spec.mole_fraction  reservoir_x_g=0.001  reservoir_y_g=0  RH_ws=1  area_A=duct_W^2 m^2
      settings: AttributesFormatString=temperature= %<reservoir_temperature>
  Controlled Heat Flow Rate Source : fl_lib/Thermal/Thermal Sources/Controlled Heat Flow Rate Source
  Coolant Properties : SimscapeFluids_lib/Thermal Liquid/Utilities/Thermal Liquid Properties (TL)  fluid_list=fluids.thermal_liquid.utilities.enum.thermal_liquid_fluid_list.ethylene_glycol  concentration_param_EG=fluids.thermal_liquid.utilities.enum.thermal_liquid_concentration.volume_fraction  concentration_param_PG=fluids.thermal_liquid.utilities.enum.thermal_liquid_concentration.volume_fraction  c_mass_SW=3.5e-3  c_mass_EG=0.1  c_mass_PG=0.1  c_mass_GL=0.1  c_vol_EG=0.5  c_vol_PG=0.1  beta_const_EG=2.1791 GPa  beta_const_PG=2.1791 GPa  beta_const_GL=2.1791 GPa  p_min_EG=0.01 MPa  p_min_PG=0.01 MPa  p_min_GL=0.01 MPa  p_max_EG=50 MPa  p_max_PG=50 MPa  p_max_GL=50 MPa  p_atm=0.101325 MPa  properties_range_check=simscape.enum.assert.action.error
  Coolant Pump : Subsystem  Tag=PublishSubsystem
      mask Display: disp(get_param(gcb, 'Name'))
  Coolant Tank : Subsystem  Tag=PublishSubsystem
      mask Display: disp(get_param(gcb, 'Name'))
  Equivalent Thermal Mass of Coolant Circuit : fl_lib/Thermal/Thermal Elements/Thermal Mass  mass_type=foundation.enum.constant_variable.constant  mass=coolant_circuit_thermal_mass kg  sp_heat=447 J/(K*kg)  mass_min=1e-6 kg  num_ports=foundation.enum.numPorts2.one  m_specify=off  m_priority=High  m=1 kg  m_nominal_specify=off  m_nominal_unit=kg  m_nominal_value=1  T_specify=on  T_priority=High  T=coolant_T_init degC  T_nominal_specify=off  T_nominal_unit=K  T_nominal_value=1  Q_specify=off  Q_priority=None  Q=0 W  Q_nominal_specify=off  Q_nominal_unit=W  Q_nominal_value=1
  Fan and Radiator : Subsystem  Variant=on  VariantControlMode=label  LabelModeActiveChoice=Fan and Radiator
      settings: PortSchema="{\"entries\":[{\"content\":{\"sides\":[{\"content\":{\"connectorIds\":[\"LConn1\",\"LConn2\",\"In1\"]},\"type\":\"ConnectorPlacement.EquallySpacedRectSide\",\"uuid\":\"87567d80-f68c-4b64-bf6a-c400b4bb513c\"},{\"content\":{\"connectorIds\":[\"Out1\",\"Out2\"],\"side\":\"RIGHT\"},\"type\":\"ConnectorPlacement.EquallySpacedRectSide\",\"uuid\":\"13164718-8307-4ae7-9828-04a93716e2b6\"},{\"content\":{\"connectorIds\":[\"LConn3\",\"LConn4\"],\"side\":\"TOP\"},\"type\":\"ConnectorPlacement.EquallySpacedRectSide\",\"uuid\":\"880ff039-95ae-477c-b44a-94cf6e1f296b\"}]},\"type\":\"ConnectorPlacement.EquallySpacedConnector\",\"uuid\":\"bcf499af-974a-4a5a-a938-12fb51c2e8c4\"}],\"packageUris\":[\"http://schema.mathworks.com/mf0/Connector/R2020b\"],\"version\":\"1.0\"}"
      mask Display: disp(get_param(gcb, 'Name'))
  Simplified Coolant circuit : SimscapeFluids_lib/Thermal Liquid/Pipes & Fittings/Pipe (TL)  dynamic_compressibility=false  inertia=false  num_segments=1  pipe_length=coolant_circuit_length m  cross_section_geometry=fluids.thermal_liquid.pipes_fittings.enum.CrossSectionGeometry.Circular  pipe_diameter=coolant_pipe_D m  pipe_inner_diameter=0.05 m  pipe_outer_diameter=0.1 m  pipe_width=0.1 m  pipe_height=0.1 m  pipe_major_axis=0.1 m  pipe_minor_axis=0.05 m  pipe_side=0.1 m  pipe_angle=30 deg  area=0.01 m^2  Dh=0.1128 m  elevation_spec=foundation.enum.constant_variable.constant  elevation_gain=0 m  gravity_spec=foundation.enum.constant_variable.constant  g=9.81 m/s^2  pressure_loss_spec=fluids.thermal_liquid.pipes_fittings.enum.PressureLossSpec.Haaland  local_pressure_loss_spec=fluids.thermal_liquid.pipes_fittings.enum.LocalLossSpec.AggregateLength  length_add=1 m  loss_coefficient=0.1  roughness_spec=fluids.thermal_liquid.pipes_fittings.enum.RoughnessSpec.CommercialPipe  roughness=15e-6 m  Re_friction_TLU=[400, 1000, 1500, 3000, 4000, 6000, 10000, 20000, 40000, 60000, 100000, 100000000]  friction_factor_TLU=[.264, .112, .071, .0417, .0387, .0268, .025, .0232, .0226, .022, .0214, .0214]  Re_lam=2000  Re_tur=4000  shape_factor=64  mdot_nominal=[.1, 1] kg/s  p_diff_nominal=[.001, .01] MPa  mdot_threshold=1e-6 kg/s  wall_spec=fluids.thermal_liquid.pipes_fittings.enum.wall_spec.rigid  vol_expansion_spec=fluids.thermal_liquid.pipes_fittings.enum.VolumeExpansionSpec.Area  area_pressure_gain=1e-6 m^2/MPa  static_pressure_TLU=[.1, 1] MPa  area_pressure_gain_TLU=[1e-05, 1.1e-05] m^2  material_behavior_spec=fluids.thermal_liquid.pipes_fittings.enum.PipeMaterialBehavior.Linear  diameter_pressure_gain=1e-6 m/MPa  wall_thickness=0.05 m  elastic_modulus=69 GPa  stress_TLU=[276, 310] MPa  strain_TLU=[.004, .02]  stress_assert_action=simscape.enum.assert.action.none  stress_max=400 MPa  poisson_ratio=0.33  wall_time_constant=0.01 s  thermal_expansion=false  alpha_L_wall=24 um/(deltaK*m)  thermal_expansion_Tref=293.15 K  heat_transfer_spec=fluids.thermal_liquid.pipes_fittings.enum.HeatTransferSpec.Gnielinski  mdot_nominal_heat=[.1, 1] kg/s  T_in_nominal=[293.15, 293.15] K  T_out_nominal=[300, 300] K  p_in_nominal_heat=[.101325, .101325] MPa  T_wall_nominal=[303.15, 303.15] K  a_coeff=0.023  b_Re_power=0.8  c_Pr_power=0.4  Nu_lam=3.66  Re_Colburn_TLU=[100, 150, 1000]  Colburn_factor_TLU=[.019, .013, .002]  Re_Nu_TLU=[100, 150, 1000]  Pr_Nu_TLU=[1, 10]  Nu_TLU=[3.72, 4.21; 3.75, 4.44; 4.21, 7.15]  p0_vec=coolant_p_init MPa  T0_vec=coolant_T_init degC  mdot0=0.1 kg/s
  Simulink-PS Converter : nesl_utility/Simulink-PS Converter  PhysicalDomain=network_engine_domain  SubClassName=ps_input  LeftPortType=input  RightPortType=output  PseudoPeriodic=off  Frequencies=[]  NoiseDistribution=none  NoiseParameters=[]  Unit=kW  AffineConversion=off  FilteringAndDerivatives=filter  SimscapeFilterOrder=1  InputFilterTimeConstant=1  UdotUserProvided=0
  Thermal Reference : fl_lib/Thermal/Thermal Elements/Thermal Reference
  A : PMIOPort  Side=Left
  B : PMIOPort  Port=2  Side=Left
  Temperature [degC] : Outport
  Pump Power [kW] : Outport  Port=2
  Radiator Fan Pwr [kW] : Outport  Port=3
  Radiator Heat Rate [kW] : Outport  Port=4
  wires:
  Coolant Pump/1(Power [kW]) -> Pump Power [kW]/1
  Coolant Pump On/Off/1 -> Coolant Pump/1(Pump ON/OFF)
  Heat flow rate [kW]/1 -> Simulink-PS Converter/1
  Radiator Fan On/Off/1 -> Fan and Radiator/1(Fan cmd)
  Fan and Radiator/1(Heat rate [kW]) -> Radiator Fan Pwr [kW]/1
  Fan and Radiator/2(Power [kW]) -> Radiator Heat Rate [kW]/1
  Coolant Tank/1(Temperature [degC]) -> Temperature [degC]/1
  connections:
  Coolant Properties/RConn1 -- Fan and Radiator/LConn2 -- B/RConn1
  Coolant Pump/RConn1 -- Simplified Coolant circuit/LConn1
  Controlled Heat Flow Rate Source/LConn1 -- Equivalent Thermal Mass of Coolant Circuit/LConn1 -- Simplified Coolant circuit/LConn2
  Thermal Reference/LConn1 -- Controlled Heat Flow Rate Source/RConn2
  Simulink-PS Converter/RConn1 -- Controlled Heat Flow Rate Source/RConn1
  Fan and Radiator/LConn3 -- Air In/LConn1
  Fan and Radiator/LConn4 -- Air Out/LConn1
  Coolant Tank/RConn1 -- Coolant Pump/LConn1
  A/RConn1 -- Coolant Tank/LConn1
  Fan and Radiator/LConn1 -- Simplified Coolant circuit/RConn1

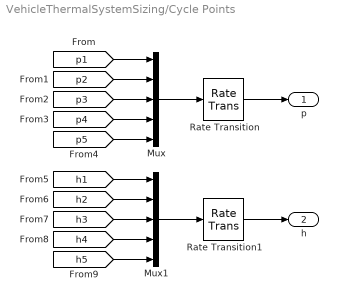
== system VehicleThermalSystemSizing/Cycle Points ==
  Mux : Mux  Inputs=5
  Mux1 : Mux  Inputs=5
  Rate Transition : RateTransition  OutPortSampleTime=10
  Rate Transition1 : RateTransition  OutPortSampleTime=10
  p : Outport
  h : Outport  Port=2
  wires:
  [p1] -> Mux/1
  [p2] -> Mux/2
  [p3] -> Mux/3
  [p4] -> Mux/4
  [p5] -> Mux/5
  Mux/1 -> Rate Transition/1
  Mux1/1 -> Rate Transition1/1
  [h5] -> Mux1/5
  [h4] -> Mux1/4
  [h3] -> Mux1/3
  [h2] -> Mux1/2
  [h1] -> Mux1/1
  Rate Transition/1 -> p/1
  Rate Transition1/1 -> h/1

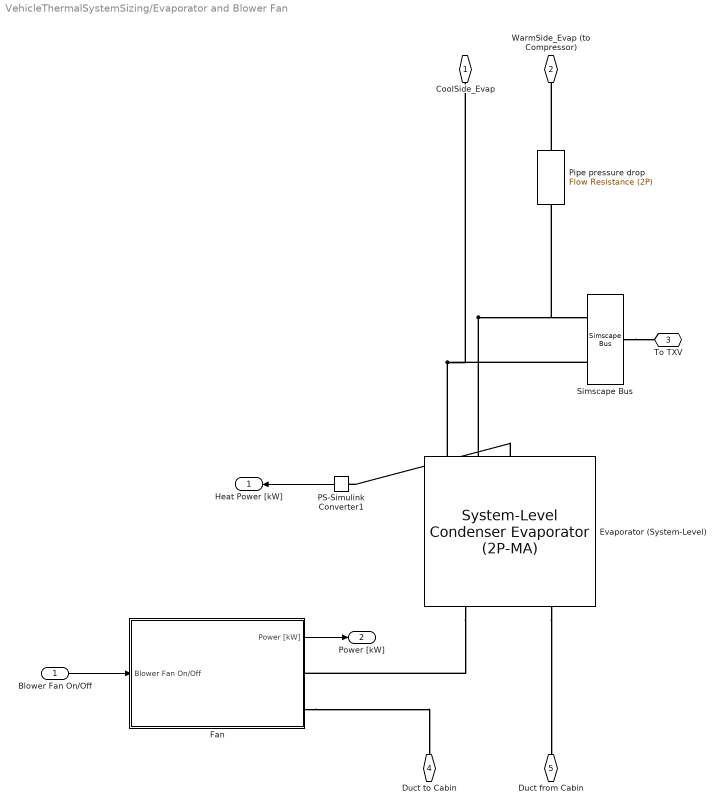
== system VehicleThermalSystemSizing/Evaporator and Blower Fan ==
  Blower Fan On/Off : Inport
  " Evaporator (System-Level)" : SimscapeFluids_lib/Fluid Network Interfaces/Heat Exchangers/System-Level Condenser Evaporator (2P-MA)  flow_arrangement=fluids.interfaces.heat_exchangers.enum.SystemLevelFlowArrangement2PMA.Cross  wall_thermal_mass=simscape.enum.onoff.off  mass_wall=1 kg  cp_wall=490 J/(K*kg)  nominal_init_wall=true  T_wall_init=293.15 K  area_A1=pi*tube_D^2/4 m^2  area_B1=pi*tube_D^2/4 m^2  area_A2=duct_W^2 m^2  area_B2=duct_W^2 m^2  operating_condition_2P=fluids.interfaces.heat_exchangers.enum.SystemLevelOperatingCondition2PMA.Evaporator  mdot_nominal_2P=0.5*refrigerant_massflowrate kg/s  delta_p_nominal_2P=0.01 MPa  pressure_spec_cond_2P=fluids.interfaces.heat_exchangers.enum.SystemLevelPressureSpecCondenser2P.InletPressure  pressure_spec_evap_2P=fluids.interfaces.heat_exchangers.enum.SystemLevelPressureSpecEvaporator2P.EvaporatingTemperature  p_in_nominal_2P=1 MPa  T_cond_nominal_2P=313.15 K  T_evap_nominal_2P=nominal_evap_temp degC  inlet_spec_2P=fluids.interfaces.heat_exchangers.enum.SystemLevelInletSpec2P.Enthalpy  T_in_nominal_2P=333.15 K  h_in_nominal_2P=evap_inlet_enthalpy kJ/kg  x_in_nominal_2P=1  capacity_spec_2P=fluids.interfaces.heat_exchangers.enum.SystemLevelCapacitySpec.OutletCondition  Q_nominal=0.1 kW  outlet_spec_cond_2P=fluids.interfaces.heat_exchangers.enum.SystemLevelOutletSpecCondenser2P.Enthalpy  outlet_spec_evap_2P=fluids.interfaces.heat_exchangers.enum.SystemLevelOutletSpecEvaporator2P.Superheating  delta_T_sub_nominal_2P=5 deltaK  delta_T_sup_nominal_2P=evap_superheat_temp deltaK  h_out_nominal_2P=250 kJ/kg  x_out_nominal_2P=0  volume_2P=0.001 m^3  nominal_init_2P=true  energy_spec_2P=foundation.enum.energy_spec.enthalpy  p_init_2P=evap_inlet_p MPa  T_init_2P=293.15 K  x_init_2P=0.5  alpha_init_2P=0.5  h_init_2P=evap_inlet_enthalpy kJ/kg  u_init_2P=1500 kJ/kg  mdot_nominal_MA=evap_air_massflowrate kg/s  delta_p_nominal_MA=0.001 MPa  p_in_nominal_MA=0.101325 MPa  T_in_nominal_MA=T_set degC  inlet_moisture_spec_MA=foundation.enum.moisture_spec.relative_humidity  RH_in_nominal_MA=0.5  x_w_in_nominal_MA=0.01  y_w_in_nominal_MA=0.01  HR_in_nominal_MA=0.01  inlet_trace_gas_spec_MA=foundation.enum.trace_gas_spec.mole_fraction  x_g_in_nominal_MA=0.001  y_g_in_nominal_MA=0  volume_MA=0.1 m^3  nominal_init_MA=true  p_init_MA=0.101325 MPa  T_init_MA=T_set degC  moisture_spec_MA=foundation.enum.moisture_spec.relative_humidity  RH_init_MA=0.5  x_w_init_MA=0.01  y_w_init_MA=0.01  HR_init_MA=0.01  trace_gas_spec_MA=foundation.enum.trace_gas_spec.mass_fraction  x_g_init_MA=0.001  y_g_init_MA=0.001  RH_ws_MA=1  a_liq_2P=0.023  a_mix_2P=0.005  a_vap_2P=0.023  b_2P=0.8  c_2P=0.33  a_MA=0.023  b_MA=0.8  c_MA=0.33
      settings: InternalSimscapePortConfiguration="{\"Bottom\":[],\"Left\":[{\"id\":\"A1\",\"label\":\"A1\",\"type\":\"foundation.two_phase_fluid.two_phase_fluid\"},{\"id\":\"B1\",\"label\":\"B1\",\"type\":\"foundation.two_phase_fluid.two_phase_fluid\"}],\"Right\":[{\"id\":\"A2\",\"label\":\"A2\",\"type\":\"foundation.moist_air.moist_air\"},{\"id\":\"B2\",\"label\":\"B2\",\"type\":\"foundation.moist_air.moist_air\"}],\"Top\":[{\"id\":\"Q1\",\"label\":\"Q1\",\"type\":\"output\"},{\"id\":\"Q2\",\"label\":\"Q2\",\"type\":\"output\"},{\"id\":\"W\",\"label\":\"W\",\"type\":\"output\"}]}"
  Fan : Subsystem  Variant=on  VariantControlMode=label  LabelModeActiveChoice=Fan_simple
  PS-Simulink Converter1 : nesl_utility/PS-Simulink Converter  PhysicalDomain=network_engine_domain  SubClassName=ps_output  LeftPortType=input  RightPortType=output  PseudoPeriodic=off  Frequencies=[]  VectorFormat=inherit  Unit=kW  AffineConversion=off
  Pipe pressure drop : fl_lib/Two-Phase Fluid/Elements/Flow Resistance (2P)  delta_p_nominal=100 Pa  mdot_nominal=refrigerant_massflowrate kg/s  v_nominal=0 m^3/kg  area=pi*tube_D^2/4 m^2  laminar_fraction=1e-3
      settings: InternalSimscapePortConfiguration="{\"Bottom\":[],\"Left\":[{\"id\":\"A\",\"label\":\"A\",\"type\":\"foundation.two_phase_fluid.two_phase_fluid\"}],\"Right\":[{\"id\":\"B\",\"label\":\"B\",\"type\":\"foundation.two_phase_fluid.two_phase_fluid\"}],\"Top\":[]}"
  Simscape Bus : SimscapeBus  HierarchyStrings=bulb;inlet
  CoolSide_Evap : PMIOPort  Side=Left
  WarmSide_Evap (to Compressor) : PMIOPort  Port=2  Side=Left
  To TXV : PMIOPort  Port=3  Side=Left
  Duct to Cabin : PMIOPort  Port=4  Side=Right
  Duct from Cabin : PMIOPort  Port=5  Side=Right
  Heat Power [kW] : Outport
  Power [kW] : Outport  Port=2
  wires:
  Blower Fan On/Off/1 -> Fan/1(Blower Fan On/Off)
  Fan/1(Power [kW]) -> Power [kW]/1
  PS-Simulink Converter1/1 -> Heat Power [kW]/1
  connections:
  " Evaporator (System-Level)"/LConn3 -- PS-Simulink Converter1/LConn1
  " Evaporator (System-Level)"/LConn1 -- Simscape Bus/LConn2 -- CoolSide_Evap/RConn1
  " Evaporator (System-Level)"/LConn2 -- Simscape Bus/LConn1 -- Pipe pressure drop/LConn1
  " Evaporator (System-Level)"/RConn2 -- Duct from Cabin/RConn1
  " Evaporator (System-Level)"/RConn1 -- Fan/RConn1
  Fan/RConn2 -- Duct to Cabin/RConn1
  Simscape Bus/RConn1 -- To TXV/RConn1
  Pipe pressure drop/RConn1 -- WarmSide_Evap (to Compressor)/RConn1

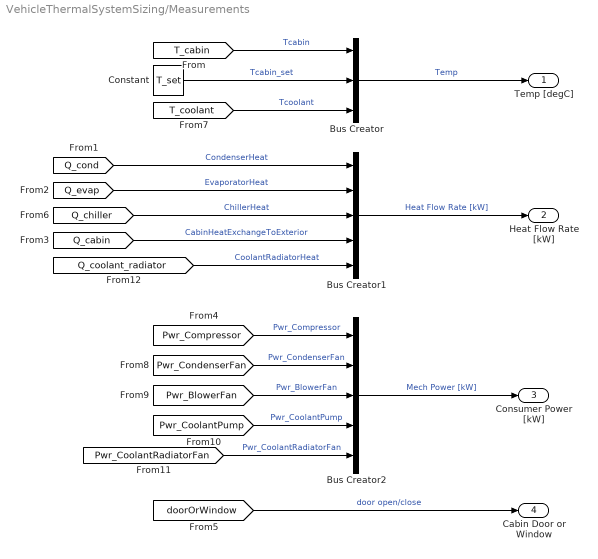
== system VehicleThermalSystemSizing/Measurements ==
  Bus Creator : BusCreator  Inputs=3
  Bus Creator1 : BusCreator  Inputs=5
  Bus Creator2 : BusCreator  Inputs=5
  Constant : Constant  Value=T_set
  Temp [degC] : Outport
  Heat Flow Rate [kW] : Outport  Port=2
  Consumer Power [kW] : Outport  Port=3
  Cabin Door or Window : Outport  Port=4
  wires:
  [T_cabin] -> Bus Creator/1  "Tcabin"
  Constant/1 -> Bus Creator/2  "Tcabin_set"
  Bus Creator/1 -> Temp [degC]/1  "Temp"
  Bus Creator1/1 -> Heat Flow Rate [kW]/1  "Heat Flow Rate [kW]"
  [Q_cond] -> Bus Creator1/1  "CondenserHeat"
  [Q_evap] -> Bus Creator1/2  "EvaporatorHeat"
  [Q_cabin] -> Bus Creator1/4  "CabinHeatExchangeToExterior"
  [doorOrWindow] -> Cabin Door or Window/1  "door open/close"
  [Q_chiller] -> Bus Creator1/3  "ChillerHeat"
  [T_coolant] -> Bus Creator/3  "Tcoolant"
  [Pwr_Compressor] -> Bus Creator2/1  "Pwr_Compressor"
  Bus Creator2/1 -> Consumer Power [kW]/1  "Mech Power [kW]"
  [Pwr_CondenserFan] -> Bus Creator2/2  "Pwr_CondenserFan"
  [Pwr_BlowerFan] -> Bus Creator2/3  "Pwr_BlowerFan"
  [Pwr_CoolantPump] -> Bus Creator2/4  "Pwr_CoolantPump"
  [Pwr_CoolantRadiatorFan] -> Bus Creator2/5  "Pwr_CoolantRadiatorFan"
  [Q_coolant_radiator] -> Bus Creator1/5  "CoolantRadiatorHeat"

== system VehicleThermalSystemSizing/Refrigerant Tank ==
  Cap (2P) : fl_lib/Two-Phase Fluid/Elements/Cap (2P)  p_specify=off  p_priority=None  p=0.101325 MPa  p_nominal_specify=off  p_nominal_unit=MPa  p_nominal_value=1  u_specify=off  u_priority=None  u=1500 kJ/kg  u_nominal_specify=off  u_nominal_unit=kJ/kg  u_nominal_value=1
      settings: InternalSimscapePortConfiguration="{\"Bottom\":[],\"Left\":[{\"id\":\"A\",\"label\":\"\",\"type\":\"foundation.two_phase_fluid.two_phase_fluid\"}],\"Right\":[],\"Top\":[]}"
  Cap (2P)1 : fl_lib/Two-Phase Fluid/Elements/Cap (2P)  p_specify=off  p_priority=None  p=0.101325 MPa  p_nominal_specify=off  p_nominal_unit=MPa  p_nominal_value=1  u_specify=off  u_priority=None  u=1500 kJ/kg  u_nominal_specify=off  u_nominal_unit=kJ/kg  u_nominal_value=1
      settings: InternalSimscapePortConfiguration="{\"Bottom\":[],\"Left\":[{\"id\":\"A\",\"label\":\"\",\"type\":\"foundation.two_phase_fluid.two_phase_fluid\"}],\"Right\":[],\"Top\":[]}"
  Coolant Reservoir : SimscapeFluids_lib/Two-Phase Fluid/Tanks & Accumulators/Receiver Accumulator (2P)  volume=pi*0.15^2/4 * 0.5 m^3  tank_area=pi*0.15^2/4 m^2  area_AV=pi*tube_D^2/4 m^2  area_BV=pi*tube_D^2/4 m^2  area_AL=pi*tube_D^2/4 m^2  area_BL=pi*tube_D^2/4 m^2  V_frac_error=simscape.enum.assert.action.none  V_frac_min=0.05  V_frac_max=0.95  V_frac_smooth=0.05  p_crit_error=simscape.enum.assert.action.error  hc_vap=20 W/(K*m^2)  hc_liq=100 W/(K*m^2)  receiver_accumulator_energy_spec=fluids.two_phase_fluid.enum.receiver_accumulator_energy_spec.enthalpy  p_init=evap_inlet_p MPa  T_init=refrig_T_init degC  M_frac_init=refrigerant_alpha_init  V_frac_init=0.5  h_init=evap_inlet_enthalpy kJ/kg  u_init=1500 kJ/kg  tau_vap_cond=1 s
      settings: InternalSimscapePortConfiguration="{\"Bottom\":[],\"Left\":[{\"id\":\"AV\",\"label\":\"AV\",\"type\":\"foundation.two_phase_fluid.two_phase_fluid\"},{\"id\":\"AL\",\"label\":\"AL\",\"type\":\"foundation.two_phase_fluid.two_phase_fluid\"},{\"id\":\"H\",\"label\":\"H\",\"type\":\"foundation.thermal.thermal\"}],\"Right\":[{\"id\":\"BV\",\"label\":\"BV\",\"type\":\"foundation.two_phase_fluid.two_phase_fluid\"},{\"id\":\"BL\",\"label\":\"BL\",\"type\":\"foundation.two_phase_fluid.two_phase_fluid\"},{\"id\":\"L\",\"label\":\"L\",\"type\":\"output\"}],\"Top\":[]}"
  Flow Resistance : fl_lib/Two-Phase Fluid/Elements/Flow Resistance (2P)  delta_p_nominal=200 Pa  mdot_nominal=refrigerant_massflowrate kg/s  v_nominal=0 m^3/kg  area=pi*tube_D^2/4 m^2  laminar_fraction=1e-3
      settings: InternalSimscapePortConfiguration="{\"Bottom\":[],\"Left\":[{\"id\":\"A\",\"label\":\"A\",\"type\":\"foundation.two_phase_fluid.two_phase_fluid\"}],\"Right\":[{\"id\":\"B\",\"label\":\"B\",\"type\":\"foundation.two_phase_fluid.two_phase_fluid\"}],\"Top\":[]}"
  Perfect Insulator : fl_lib/Thermal/Thermal Elements/Perfect Insulator  T_specify=off  T_priority=None  T=293.15 K  T_nominal_specify=off  T_nominal_unit=K  T_nominal_value=1
  A : PMIOPort  Side=Left
  B : PMIOPort  Port=2  Side=Right
  connections:
  Perfect Insulator/LConn1 -- Coolant Reservoir/LConn3
  Cap (2P)1/LConn1 -- Coolant Reservoir/LConn1
  Cap (2P)/LConn1 -- Coolant Reservoir/RConn1
  Coolant Reservoir/RConn2 -- Flow Resistance/LConn1
  A/RConn1 -- Coolant Reservoir/LConn2
  Flow Resistance/RConn1 -- B/RConn1
